simulink model "week1_5"  (R2020b)
settings: Solver=VariableStepAuto  StartTime=0.0  StopTime=10.0  RelTol=1e-3
model workspace (MAT data in the model file):
  C = Simulink.Parameter
  C.Value = 0.001
  C.DataType = 'auto'
  C.Dimensions = [1 1]
  R = Simulink.Parameter
  R.Value = 10
  R.DataType = 'auto'
  R.Dimensions = [1 1]
libraries: simulink x1
settings Model: Creator=Lenovo  LastModifiedBy=Lenovo

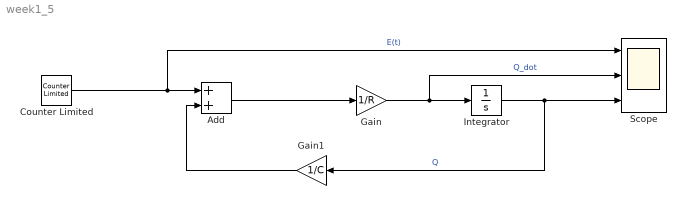
== system week1_5 ==
  Add : Sum
  Counter Limited : simulink/Sources/Counter Limited  uplimit=7  tsamp=-1
  Gain : Gain  Gain=1/R
  Gain1 : Gain  Gain=1/C
  Integrator : Integrator
  Scope : Scope  NumInputPorts=3
  wires:
  Counter Limited/1 -> Scope/1, Add/1  "E(t)"
  Add/1 -> Gain/1
  Gain/1 -> Scope/2, Integrator/1  "Q_dot"
  Integrator/1 -> Gain1/1, Scope/3  "Q"
  Gain1/1 -> Add/2
